simulink model "p9_Sim_Transfer_Func_Diagram"  (R2017b)
settings: Solver=ode14x  StartTime=0.0  StopTime=3  FixedStep=.001  RelTol=1e-3
settings Model: Creator=Harrison  LastModifiedBy=Harrison
settings DataIOCC: SaveFormat=Array

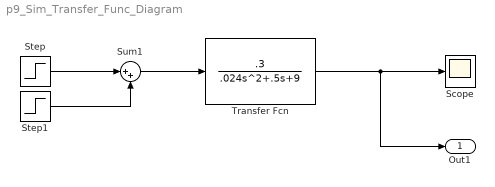
== system p9_Sim_Transfer_Func_Diagram ==
  Scope : Scope
  Step : Step  Time=0  After=10  SampleTime=0
  Step1 : Step  Time=.1  After=-10  SampleTime=0
  Sum1 : Sum  Inputs=|++
  Transfer Fcn : TransferFcn  Numerator=[.3]  Denominator=[.024 .5 9]
  Out1 : Outport
  wires:
  Step/1 -> Sum1/1
  Step1/1 -> Sum1/2
  Sum1/1 -> Transfer Fcn/1
  Transfer Fcn/1 -> Out1/1, Scope/1
